simulink model "ysw3_41"  (R2014a)
settings: Solver=ode45  StartTime=0.0  StopTime=10.0  RelTol=1e-3
settings Model: Creator=Administrator  LastModifiedBy=Administrator

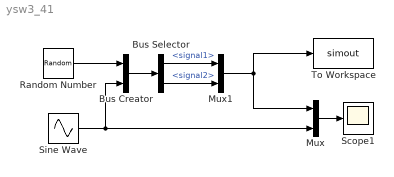
== system ysw3_41 ==
  Bus Creator : BusCreator  Inputs=2
  Bus Selector : BusSelector  OutputSignals=signal1,signal2
  Mux : Mux  Inputs=2
  Mux1 : Mux  Inputs=2
  Random Number : RandomNumber  SampleTime=0.1
  Scope1 : Scope
      settings: TimeRange=10
  Sine Wave : Sin  SampleTime=0.1
  To Workspace : ToWorkspace  VariableName=simout  SaveFormat=Timeseries  SampleTime=-1
  wires:
  Mux/1 -> Scope1/1
  Sine Wave/1 -> Bus Creator/2, Mux/2
  Mux1/1 -> Mux/1, To Workspace/1
  Random Number/1 -> Bus Creator/1
  Bus Creator/1 -> Bus Selector/1
  Bus Selector/1 -> Mux1/1  "<signal1>"
  Bus Selector/2 -> Mux1/2  "<signal2>"
